simulink subsystem "Kinematika_A"  (R2024b)
settings: Solver=VariableStepAuto  StartTime=0.0  StopTime=10.0  RelTol=1e-3
values from neighbouring files (symbols this model uses):
  L = 0.15    [D1script.m]    (also in disp.mat = 0.1; onlabscript.m = 0.1)
  R = 0.05    [D1script.m]    (also in disp.mat = 0.02; onlabscript.m = 0.02)
settings Model: Creator=Asus  LastModifiedBy=Asus

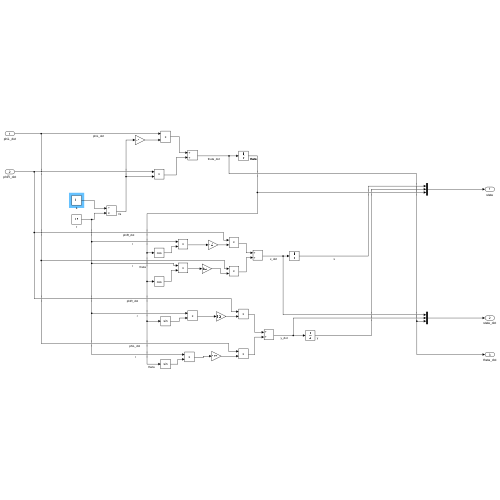
[thumbnail: Simulink's stored preview of the top-level diagram]
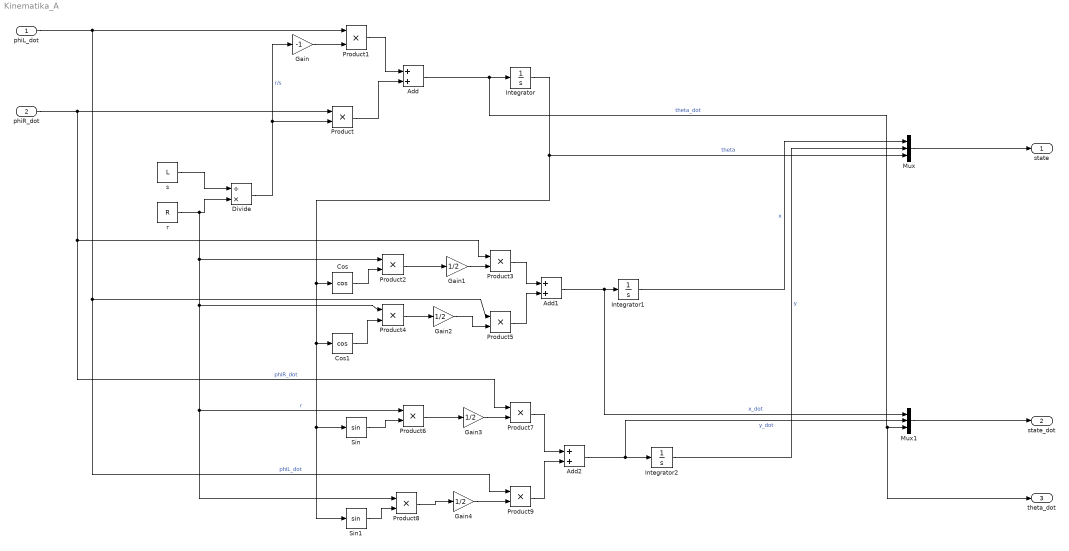
== system Kinematika_A ==
  phiL_dot : Inport
  phiR_dot : Inport  Port=2
  Add : Sum
  Add1 : Sum
  Add2 : Sum
  Cos : Trigonometry  Operator=cos
  Cos1 : Trigonometry  Operator=cos
  Divide : Product  Inputs=/*
  Gain : Gain  Gain=-1
  Gain{1..4} (4 alike) : Gain  Gain=1/2
  Integrator : Integrator
  Integrator1 : Integrator
  Integrator2 : Integrator
  Mux : Mux  Inputs=3
  Mux1 : Mux  Inputs=3
  Product{,1..9} (10 alike) : Product
  Sin : Trigonometry
  Sin1 : Trigonometry
  r : Constant  Value=R
  s : Constant  Value=L
  state : Outport
  state_dot : Outport  Port=2
  theta_dot : Outport  Port=3
  wires:
  s/1 -> Divide/1
  Gain/1 -> Product1/2
  phiL_dot/1 -> Product5/1, Product9/1, Product1/1  "phiL_dot"
  Divide/1 -> Gain/1, Product/2  "r/s"
  phiR_dot/1 -> Product3/1, Product7/1, Product/1  "phiR_dot"
  Product1/1 -> Add/1
  Product/1 -> Add/2
  Add/1 -> Integrator/1, Mux1/3, theta_dot/1  "theta_dot"
  Integrator/1 -> Cos/1, Cos1/1, Sin/1, Sin1/1, Mux/3  "theta"
  Cos/1 -> Product2/2
  Product2/1 -> Gain1/1
  Gain1/1 -> Product3/2
  Product4/1 -> Gain2/1
  Gain2/1 -> Product5/2
  Cos1/1 -> Product4/2
  r/1 -> Divide/2, Product2/1, Product4/1, Product6/1, Product8/1  "r"
  Product3/1 -> Add1/1
  Product5/1 -> Add1/2
  Add1/1 -> Integrator1/1, Mux1/1  "x_dot"
  Integrator1/1 -> Mux/1  "x"
  Sin/1 -> Product6/2
  Product6/1 -> Gain3/1
  Gain3/1 -> Product7/2
  Sin1/1 -> Product8/2
  Product8/1 -> Gain4/1
  Gain4/1 -> Product9/2
  Product9/1 -> Add2/2
  Product7/1 -> Add2/1
  Add2/1 -> Integrator2/1, Mux1/2  "y_dot"
  Integrator2/1 -> Mux/2  "y"
  Mux/1 -> state/1
  Mux1/1 -> state_dot/1
